simulink model "drivingDistance"  (R2017b)
settings: Solver=VariableStepAuto  StartTime=0.0  StopTime=10.0  RelTol=1e-3
settings Model: Creator=frank  LastModifiedBy=frank

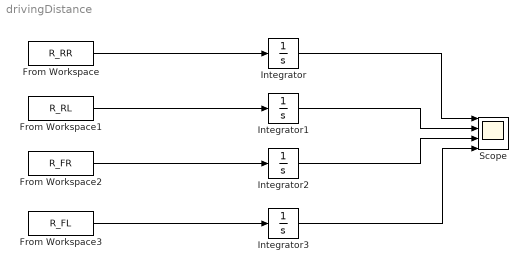
== system drivingDistance ==
  From Workspace : FromWorkspace  VariableName=R_RR  SampleTime=0
  From Workspace1 : FromWorkspace  VariableName=R_RL  SampleTime=0
  From Workspace2 : FromWorkspace  VariableName=R_FR  SampleTime=0
  From Workspace3 : FromWorkspace  VariableName=R_FL  SampleTime=0
  Integrator{,1..3} (4 alike) : Integrator
  Scope : Scope  NumInputPorts=4
  wires:
  From Workspace/1 -> Integrator/1
  From Workspace1/1 -> Integrator1/1
  From Workspace2/1 -> Integrator2/1
  From Workspace3/1 -> Integrator3/1
  Integrator/1 -> Scope/1
  Integrator1/1 -> Scope/2
  Integrator2/1 -> Scope/3
  Integrator3/1 -> Scope/4
